simulink model "pendule_inv_capteur_etu"  (R2023a)
settings: Solver=ode4  StartTime=0.0  StopTime=100.0  RelTol=1e-3
values from neighbouring files (symbols this model uses):
  g = 9.81    [init.m]
  K = [30 10]    [init.m]
  l = 10    [init.m]
  ue = 0    [init.m]
  x0 = [pi/20 0]'    [init.m]
  xe = [0 0]'    [init.m]
settings Model: Creator=fhudrisi  LastModifiedBy=ymeziani
settings OptimizationCC: ReuseModelBlockBuffer=off
settings DebuggingCC: UnconnectedInputMsg=warning  UnconnectedOutputMsg=warning  UnconnectedLineMsg=warning
settings ModelReferenceCC: EnableRefExpFcnMdlSchedulingChecks=on
settings RTWCC: DLArmComputeVersion=19.05

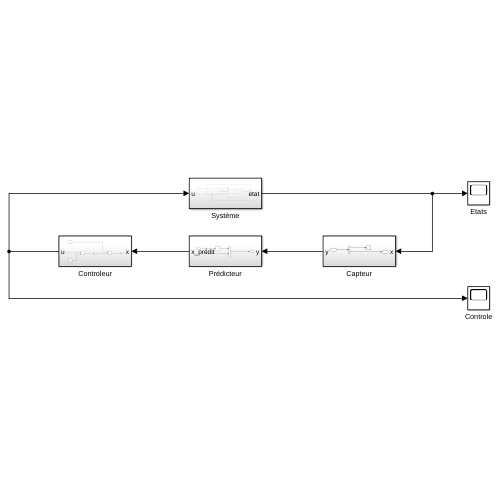
[thumbnail: Simulink's stored preview of the top-level diagram]
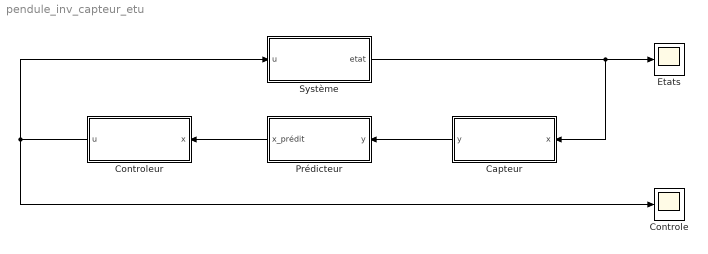
== system pendule_inv_capteur_etu ==
  Capteur : Subsystem
  Controle : Scope
  Controleur : Subsystem
  Etats : Scope
  Prédicteur : Subsystem
  Système : Subsystem
  wires:
  Système/1(etat) -> Etats/1, Capteur/1(x)
  Controleur/1(u) -> Controle/1, Système/1(u)
  Capteur/1(y) -> Prédicteur/1(y)
  Prédicteur/1(x_prédit) -> Controleur/1(x)

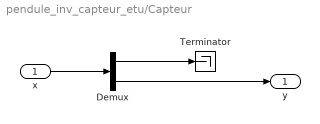
== system pendule_inv_capteur_etu/Capteur ==
  x : Inport
  Demux : Demux  Outputs=2
  Terminator : Terminator
  y : Outport
  wires:
  x/1 -> Demux/1
  Demux/2 -> y/1
  Demux/1 -> Terminator/1

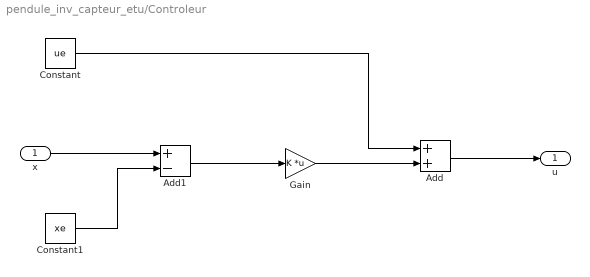
== system pendule_inv_capteur_etu/Controleur ==
  x : Inport
  Add : Sum
  Add1 : Sum  Inputs=+-
  Constant : Constant  Value=ue
  Constant1 : Constant  Value=xe
  Gain : Gain  Gain=K  Multiplication=Matrix(K*u)
  u : Outport
  wires:
  Constant1/1 -> Add1/2
  Gain/1 -> Add/2
  Add/1 -> u/1
  Constant/1 -> Add/1
  Add1/1 -> Gain/1
  x/1 -> Add1/1

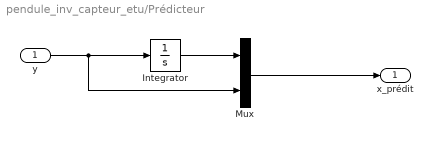
== system pendule_inv_capteur_etu/Prédicteur ==
  y : Inport
  Integrator : Integrator  InitialCondition=x0(1)
  Mux : Mux  Inputs=2
  x_prédit : Outport
  wires:
  y/1 -> Mux/2, Integrator/1
  Integrator/1 -> Mux/1
  Mux/1 -> x_prédit/1

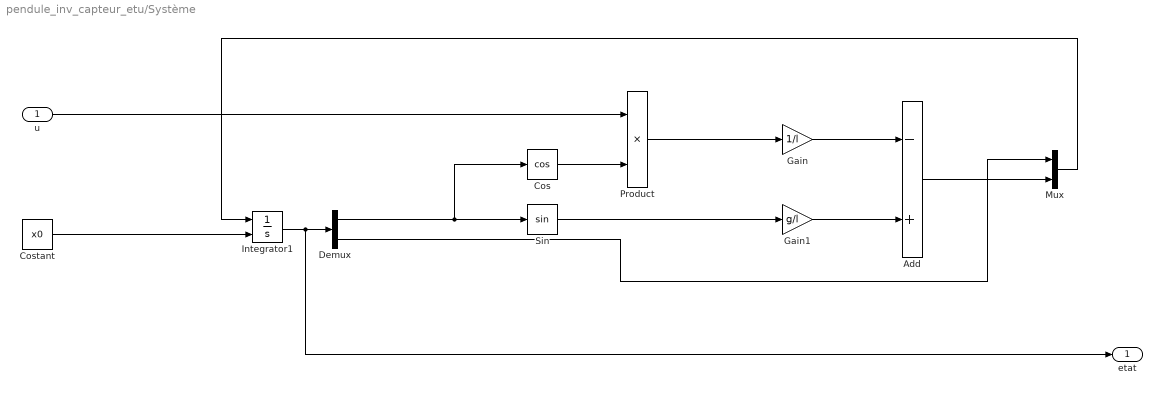
== system pendule_inv_capteur_etu/Système ==
  u : Inport
  Add : Sum  Inputs=-+
  Cos : Trigonometry  Operator=cos
  Costant : Constant  Value=x0
  Demux : Demux  Outputs=2
  Gain : Gain  Gain=1/l
  Gain1 : Gain  Gain=g/l
  Integrator1 : Integrator  InitialConditionSource=external
  Mux : Mux  Inputs=2
  Product : Product
  Sin : Trigonometry
  etat : Outport
  wires:
  Add/1 -> Mux/2
  Mux/1 -> Integrator1/1
  Integrator1/1 -> etat/1, Demux/1
  Demux/1 -> Sin/1, Cos/1
  u/1 -> Product/1
  Sin/1 -> Gain1/1
  Costant/1 -> Integrator1/2
  Cos/1 -> Product/2
  Product/1 -> Gain/1
  Demux/2 -> Mux/1
  Gain1/1 -> Add/2
  Gain/1 -> Add/1
